simulink model "env_pid"  (R2024b)
settings: Solver=VariableStepAuto  StartTime=0.0  StopTime=1000  RelTol=1e-3  AbsTol=1e-3  EnableMultiTasking=on
PreLoadFcn:
  | inertiaDriveShaft = 12;
  | ratioDiff = 2;
  | radiusWheel = 16*2.54/100;
  | massVehicle = 1500;
  | inertiaLateral = 25*(radiusWheel)^2;
  | beta = 15;
  | engineRPM0 = 800;
  | tireStiffness = 200000;
  | tireDamping = 1000;
  | 
  | Simple=Simulink.VariantExpression('TIRE==1');
  | Friction=Simulink.VariantExpression('TIRE==2');
  | MFormula=Simulink.VariantExpression('TIRE==3');
  | 
  | TIRE=3;
model workspace (MAT data in the model file):
  Beta = -10
  Toque1 = 0
  Toque_f = 0
  Toque_r = 100
  Torque_f = 0
  Torque_r = 0
libraries: sdl_lib x18, nesl_utility x10, fl_lib x4, fl_ps_legacy_lib x4, slpidlib x1
(part 6 of 6)

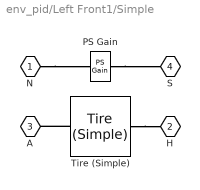
== system env_pid/Left Front1/Simple ==
  PS Gain : fl_ps_legacy_lib/Legacy Physical Signals/Functions/PS Gain  gain=0
  Tire (Simple) : sdl_lib/Tires & Vehicles/Tire (Simple)  r_tire=radiusWheel m  model_compliance=1  stiffness=tireStiffness N/m  damping=tireDamping N/(m/s)  model_inertia=1  tire_inertia=inertiaLateral/2 kg*m^2  initial_velocity=0 rpm
      settings: InternalSimscapePortConfiguration="{\"Bottom\":[],\"Left\":[{\"id\":\"A\",\"label\":\"A\",\"type\":\"foundation.mechanical.rotational.rotational\"}],\"Right\":[{\"id\":\"H\",\"label\":\"H\",\"type\":\"foundation.mechanical.translational.translational\"}],\"Top\":[]}"
  N : PMIOPort  Side=Left
  H : PMIOPort  Port=2  Side=Left
  A : PMIOPort  Port=3  Side=Left
  S : PMIOPort  Port=4  Side=Right
  connections:
  Tire (Simple)/LConn1 -- A/RConn1
  Tire (Simple)/RConn1 -- H/RConn1
  N/RConn1 -- PS Gain/LConn1
  PS Gain/RConn1 -- S/RConn1

== system env_pid/Left Rear1/Friction Parameterized ==
  Tire (Friction Parameterized) : sdl_lib/Tires & Vehicles/Tire (Friction Parameterized)  r_tire=radiusWheel m  slip_output=sdl.enum.SlipOutput.Relative  friction_model=sdl.enum.friction_model_var.fixed  mu_static=0.9  mu_kinetic=0.7  slip_vector=-flip([ 0 0.02 0.06 0.15 0.6 1 ]) rad/s  mu_kinetic_vector=flip([ 0.89 0.88 0.8 0.75 0.7 0.7 ])  interp_method=simscape.enum.interpolation.linear  extrap_method=simscape.enum.extrapolation.linear  model_compliance=1  stiffness=tireStiffness N/m  damping=tireDamping N/(m/s)  model_inertia=1  wheel_inertia=0.7*(inertiaLateral/2) kg*m^2  belt_inertia=0.3*(inertiaLateral/2) kg*m^2  initial_velocity=0 rpm  model_resistance=1  resistance_model=2  coeff=0.015  p_tire=250e3 Pa  alpha=-0.003  beta=0.97  coeff_a=84e-4  coeff_b=6.2e-4 s/m  coeff_c=1.6e-4 s^2/m^2  v_thr=1e-3 m/s  v_tol=0.01 m/s  F_min=10 N  initial_traction_state=1
      settings: InternalSimscapePortConfiguration="{\"Bottom\":[],\"Left\":[{\"id\":\"N\",\"label\":\"N\",\"type\":\"input\"},{\"id\":\"A\",\"label\":\"A\",\"type\":\"foundation.mechanical.rotational.rotational\"}],\"Right\":[{\"id\":\"Srel\",\"label\":\"S\",\"type\":\"output\"},{\"id\":\"H\",\"label\":\"H\",\"type\":\"foundation.mechanical.translational.translational\"}],\"Top\":[]}"
  N : PMIOPort  Side=Left
  H : PMIOPort  Port=2  Side=Left
  A : PMIOPort  Port=3  Side=Left
  S : PMIOPort  Port=4  Side=Right
  connections:
  Tire (Friction Parameterized)/LConn2 -- A/RConn1
  Tire (Friction Parameterized)/LConn1 -- N/RConn1
  Tire (Friction Parameterized)/RConn2 -- H/RConn1
  Tire (Friction Parameterized)/RConn1 -- S/RConn1

== system env_pid/Left Rear1/Magic Formula ==
  Tire (Magic Formula) : sdl_lib/Tires & Vehicles/Tire (Magic Formula)  parameterization=1  F_z1=3000 N  F_x1=3500 N  kappa1=10  B_m=10  C_m=1.9  D_m=1  E_m=0.97  fz0=4e+3 N  p_Cx=1.685  p_Dx=[ 1.21 -0.037 ]  p_Ex=[ 0.344 0.095 -0.02 0 ]  p_Kx=[ 21.51 -0.163 0.245 ]  p_Hx=[ -0.002 0.002 ]  p_Vx=[ 0 0 ]  rolling_radius_model=sdl.enum.RollingRadiusParameterization.Constant  r_e=radiusWheel m  r_0=0.3 m  breff=8.39  dreff=0.26  freff=0.074  q_re0=0.99  q_v1=0.008  longvl=17 m/s  cz=5e5 N/m  model_resistance=1  resistance_model=1  coeff=0.015  p_tire=250e3 Pa  alpha=-0.003  beta=0.97  coeff_a=84e-4  coeff_b=6.2e-4 s/m  coeff_c=1.6e-4 s^2/m^2  p_tire0=240e3 Pa  fz0_resistance=4000 N  vH0=16 m/s  q_Sy=[.0082, 0, .0014, .001, 0, 0, 1.08, -.5]  v_thr=1e-3 m/s  enable_scaling_coefficients=false  lfzO=1  lcx=1  lmux=1  lex=1  lkx=1  lhx=1  lvx=1  lmy=1  model_compliance=1  stiffness=tireStiffness N/m  damping=tireDamping N/(m/s)  model_inertia=1  inertia=inertiaLateral/2 kg*m^2  initial_velocity=0 rpm  vxlow=0.1 m/s  v_tr_thr=0.1*(0.1) m/s  kpumin=-1e5  kpumax=1e5
  N : PMIOPort  Side=Left
  H : PMIOPort  Port=2  Side=Left
  A : PMIOPort  Port=3  Side=Left
  S : PMIOPort  Port=4  Side=Right
  connections:
  Tire (Magic Formula)/RConn1 -- S/RConn1
  Tire (Magic Formula)/RConn2 -- H/RConn1
  Tire (Magic Formula)/LConn1 -- N/RConn1
  Tire (Magic Formula)/LConn2 -- A/RConn1

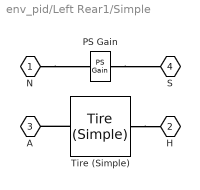
== system env_pid/Left Rear1/Simple ==
  PS Gain : fl_ps_legacy_lib/Legacy Physical Signals/Functions/PS Gain  gain=0
  Tire (Simple) : sdl_lib/Tires & Vehicles/Tire (Simple)  r_tire=radiusWheel m  model_compliance=1  stiffness=tireStiffness N/m  damping=tireDamping N/(m/s)  model_inertia=1  tire_inertia=inertiaLateral/2 kg*m^2  initial_velocity=0 rpm
      settings: InternalSimscapePortConfiguration="{\"Bottom\":[],\"Left\":[{\"id\":\"A\",\"label\":\"A\",\"type\":\"foundation.mechanical.rotational.rotational\"}],\"Right\":[{\"id\":\"H\",\"label\":\"H\",\"type\":\"foundation.mechanical.translational.translational\"}],\"Top\":[]}"
  N : PMIOPort  Side=Left
  H : PMIOPort  Port=2  Side=Left
  A : PMIOPort  Port=3  Side=Left
  S : PMIOPort  Port=4  Side=Right
  connections:
  PS Gain/RConn1 -- S/RConn1
  N/RConn1 -- PS Gain/LConn1
  Tire (Simple)/RConn1 -- H/RConn1
  Tire (Simple)/LConn1 -- A/RConn1

== system env_pid/Right Front1/Friction Parameterized ==
  Tire (Friction Parameterized) : sdl_lib/Tires & Vehicles/Tire (Friction Parameterized)  r_tire=radiusWheel m  slip_output=sdl.enum.SlipOutput.Relative  friction_model=sdl.enum.friction_model_var.fixed  mu_static=0.9  mu_kinetic=0.7  slip_vector=-flip([ 0 0.02 0.06 0.15 0.6 1 ]) rad/s  mu_kinetic_vector=flip([ 0.89 0.88 0.8 0.75 0.7 0.7 ])  interp_method=simscape.enum.interpolation.linear  extrap_method=simscape.enum.extrapolation.linear  model_compliance=1  stiffness=tireStiffness N/m  damping=tireDamping N/(m/s)  model_inertia=1  wheel_inertia=0.7*(inertiaLateral/2) kg*m^2  belt_inertia=0.3*(inertiaLateral/2) kg*m^2  initial_velocity=0 rpm  model_resistance=1  resistance_model=2  coeff=0.015  p_tire=250e3 Pa  alpha=-0.003  beta=0.97  coeff_a=84e-4  coeff_b=6.2e-4 s/m  coeff_c=1.6e-4 s^2/m^2  v_thr=1e-3 m/s  v_tol=0.01 m/s  F_min=10 N  initial_traction_state=1
      settings: InternalSimscapePortConfiguration="{\"Bottom\":[],\"Left\":[{\"id\":\"N\",\"label\":\"N\",\"type\":\"input\"},{\"id\":\"A\",\"label\":\"A\",\"type\":\"foundation.mechanical.rotational.rotational\"}],\"Right\":[{\"id\":\"Srel\",\"label\":\"S\",\"type\":\"output\"},{\"id\":\"H\",\"label\":\"H\",\"type\":\"foundation.mechanical.translational.translational\"}],\"Top\":[]}"
  N : PMIOPort  Side=Left
  H : PMIOPort  Port=2  Side=Left
  A : PMIOPort  Port=3  Side=Left
  S : PMIOPort  Port=4  Side=Right
  connections:
  Tire (Friction Parameterized)/LConn2 -- A/RConn1
  Tire (Friction Parameterized)/LConn1 -- N/RConn1
  Tire (Friction Parameterized)/RConn2 -- H/RConn1
  Tire (Friction Parameterized)/RConn1 -- S/RConn1

== system env_pid/Right Front1/Magic Formula ==
  Tire (Magic Formula) : sdl_lib/Tires & Vehicles/Tire (Magic Formula)  parameterization=1  F_z1=3000 N  F_x1=3500 N  kappa1=10  B_m=10  C_m=1.9  D_m=1  E_m=0.97  fz0=4e+3 N  p_Cx=1.685  p_Dx=[ 1.21 -0.037 ]  p_Ex=[ 0.344 0.095 -0.02 0 ]  p_Kx=[ 21.51 -0.163 0.245 ]  p_Hx=[ -0.002 0.002 ]  p_Vx=[ 0 0 ]  rolling_radius_model=sdl.enum.RollingRadiusParameterization.Constant  r_e=radiusWheel m  r_0=0.3 m  breff=8.39  dreff=0.26  freff=0.074  q_re0=0.99  q_v1=0.008  longvl=17 m/s  cz=5e5 N/m  model_resistance=1  resistance_model=1  coeff=0.015  p_tire=250e3 Pa  alpha=-0.003  beta=0.97  coeff_a=84e-4  coeff_b=6.2e-4 s/m  coeff_c=1.6e-4 s^2/m^2  p_tire0=240e3 Pa  fz0_resistance=4000 N  vH0=16 m/s  q_Sy=[.0082, 0, .0014, .001, 0, 0, 1.08, -.5]  v_thr=1e-3 m/s  enable_scaling_coefficients=false  lfzO=1  lcx=1  lmux=1  lex=1  lkx=1  lhx=1  lvx=1  lmy=1  model_compliance=1  stiffness=tireStiffness N/m  damping=tireDamping N/(m/s)  model_inertia=1  inertia=inertiaLateral/2 kg*m^2  initial_velocity=0 rpm  vxlow=0.1 m/s  v_tr_thr=0.1*(0.1) m/s  kpumin=-1e5  kpumax=1e5
  N : PMIOPort  Side=Left
  H : PMIOPort  Port=2  Side=Left
  A : PMIOPort  Port=3  Side=Left
  S : PMIOPort  Port=4  Side=Right
  connections:
  Tire (Magic Formula)/RConn1 -- S/RConn1
  Tire (Magic Formula)/RConn2 -- H/RConn1
  Tire (Magic Formula)/LConn1 -- N/RConn1
  Tire (Magic Formula)/LConn2 -- A/RConn1

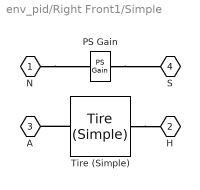
== system env_pid/Right Front1/Simple ==
  PS Gain : fl_ps_legacy_lib/Legacy Physical Signals/Functions/PS Gain  gain=0
  Tire (Simple) : sdl_lib/Tires & Vehicles/Tire (Simple)  r_tire=radiusWheel m  model_compliance=1  stiffness=tireStiffness N/m  damping=tireDamping N/(m/s)  model_inertia=1  tire_inertia=inertiaLateral/2 kg*m^2  initial_velocity=0 rpm
      settings: InternalSimscapePortConfiguration="{\"Bottom\":[],\"Left\":[{\"id\":\"A\",\"label\":\"A\",\"type\":\"foundation.mechanical.rotational.rotational\"}],\"Right\":[{\"id\":\"H\",\"label\":\"H\",\"type\":\"foundation.mechanical.translational.translational\"}],\"Top\":[]}"
  N : PMIOPort  Side=Left
  H : PMIOPort  Port=2  Side=Left
  A : PMIOPort  Port=3  Side=Left
  S : PMIOPort  Port=4  Side=Right
  connections:
  PS Gain/RConn1 -- S/RConn1
  N/RConn1 -- PS Gain/LConn1
  Tire (Simple)/RConn1 -- H/RConn1
  Tire (Simple)/LConn1 -- A/RConn1

== system env_pid/Right Rear1/Friction Parameterized ==
  Tire (Friction Parameterized) : sdl_lib/Tires & Vehicles/Tire (Friction Parameterized)  r_tire=radiusWheel m  slip_output=sdl.enum.SlipOutput.Relative  friction_model=sdl.enum.friction_model_var.fixed  mu_static=0.9  mu_kinetic=0.7  slip_vector=-flip([ 0 0.02 0.06 0.15 0.6 1 ]) rad/s  mu_kinetic_vector=flip([ 0.89 0.88 0.8 0.75 0.7 0.7 ])  interp_method=simscape.enum.interpolation.linear  extrap_method=simscape.enum.extrapolation.linear  model_compliance=1  stiffness=tireStiffness N/m  damping=tireDamping N/(m/s)  model_inertia=1  wheel_inertia=0.7*(inertiaLateral/2) kg*m^2  belt_inertia=0.3*(inertiaLateral/2) kg*m^2  initial_velocity=0 rpm  model_resistance=1  resistance_model=2  coeff=0.015  p_tire=250e3 Pa  alpha=-0.003  beta=0.97  coeff_a=84e-4  coeff_b=6.2e-4 s/m  coeff_c=1.6e-4 s^2/m^2  v_thr=1e-3 m/s  v_tol=0.01 m/s  F_min=10 N  initial_traction_state=1
      settings: InternalSimscapePortConfiguration="{\"Bottom\":[],\"Left\":[{\"id\":\"N\",\"label\":\"N\",\"type\":\"input\"},{\"id\":\"A\",\"label\":\"A\",\"type\":\"foundation.mechanical.rotational.rotational\"}],\"Right\":[{\"id\":\"Srel\",\"label\":\"S\",\"type\":\"output\"},{\"id\":\"H\",\"label\":\"H\",\"type\":\"foundation.mechanical.translational.translational\"}],\"Top\":[]}"
  N : PMIOPort  Side=Left
  H : PMIOPort  Port=2  Side=Left
  A : PMIOPort  Port=3  Side=Left
  S : PMIOPort  Port=4  Side=Right
  connections:
  Tire (Friction Parameterized)/RConn1 -- S/RConn1
  Tire (Friction Parameterized)/RConn2 -- H/RConn1
  Tire (Friction Parameterized)/LConn1 -- N/RConn1
  Tire (Friction Parameterized)/LConn2 -- A/RConn1

== system env_pid/Right Rear1/Magic Formula ==
  Tire (Magic Formula) : sdl_lib/Tires & Vehicles/Tire (Magic Formula)  parameterization=1  F_z1=3000 N  F_x1=3500 N  kappa1=10  B_m=10  C_m=1.9  D_m=1  E_m=0.97  fz0=4e+3 N  p_Cx=1.685  p_Dx=[ 1.21 -0.037 ]  p_Ex=[ 0.344 0.095 -0.02 0 ]  p_Kx=[ 21.51 -0.163 0.245 ]  p_Hx=[ -0.002 0.002 ]  p_Vx=[ 0 0 ]  rolling_radius_model=sdl.enum.RollingRadiusParameterization.Constant  r_e=radiusWheel m  r_0=0.3 m  breff=8.39  dreff=0.26  freff=0.074  q_re0=0.99  q_v1=0.008  longvl=17 m/s  cz=5e5 N/m  model_resistance=1  resistance_model=1  coeff=0.015  p_tire=250e3 Pa  alpha=-0.003  beta=0.97  coeff_a=84e-4  coeff_b=6.2e-4 s/m  coeff_c=1.6e-4 s^2/m^2  p_tire0=240e3 Pa  fz0_resistance=4000 N  vH0=16 m/s  q_Sy=[.0082, 0, .0014, .001, 0, 0, 1.08, -.5]  v_thr=1e-3 m/s  enable_scaling_coefficients=false  lfzO=1  lcx=1  lmux=1  lex=1  lkx=1  lhx=1  lvx=1  lmy=1  model_compliance=1  stiffness=tireStiffness N/m  damping=tireDamping N/(m/s)  model_inertia=1  inertia=inertiaLateral/2 kg*m^2  initial_velocity=0 rpm  vxlow=0.1 m/s  v_tr_thr=0.1*(0.1) m/s  kpumin=-1e5  kpumax=1e5
  N : PMIOPort  Side=Left
  H : PMIOPort  Port=2  Side=Left
  A : PMIOPort  Port=3  Side=Left
  S : PMIOPort  Port=4  Side=Right
  connections:
  Tire (Magic Formula)/LConn2 -- A/RConn1
  Tire (Magic Formula)/LConn1 -- N/RConn1
  Tire (Magic Formula)/RConn2 -- H/RConn1
  Tire (Magic Formula)/RConn1 -- S/RConn1

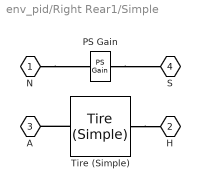
== system env_pid/Right Rear1/Simple ==
  PS Gain : fl_ps_legacy_lib/Legacy Physical Signals/Functions/PS Gain  gain=0
  Tire (Simple) : sdl_lib/Tires & Vehicles/Tire (Simple)  r_tire=radiusWheel m  model_compliance=1  stiffness=tireStiffness N/m  damping=tireDamping N/(m/s)  model_inertia=1  tire_inertia=inertiaLateral/2 kg*m^2  initial_velocity=0 rpm
      settings: InternalSimscapePortConfiguration="{\"Bottom\":[],\"Left\":[{\"id\":\"A\",\"label\":\"A\",\"type\":\"foundation.mechanical.rotational.rotational\"}],\"Right\":[{\"id\":\"H\",\"label\":\"H\",\"type\":\"foundation.mechanical.translational.translational\"}],\"Top\":[]}"
  N : PMIOPort  Side=Left
  H : PMIOPort  Port=2  Side=Left
  A : PMIOPort  Port=3  Side=Left
  S : PMIOPort  Port=4  Side=Right
  connections:
  Tire (Simple)/LConn1 -- A/RConn1
  Tire (Simple)/RConn1 -- H/RConn1
  N/RConn1 -- PS Gain/LConn1
  PS Gain/RConn1 -- S/RConn1

== matlab function env_pid/MATLAB Function ==
  data: grid input; v_x output; v input
function v_x = fcn(grid, v)
% grid = tan(θ)*100
v_x = v/sqrt(1+(grid/100)^2);
